simulink model "autoland_control"  (Simulink 8.4)
settings: Solver=FixedStepDiscrete  StartTime=0.0  StopTime=20.0  FixedStep=SampleTime  RelTol=1e-3
undefined symbols (not defined in the file or in its folder): AC, approach_sinkrate, approach_speed, autoland_flag, autothrottle_gains, engage_flare, flare_timeconstant, landing_sinkrate, landing_speed, SampleTime, sinkrate, sinkrate_gains, theta_sat, TrimCondition
libraries: Actuator_Lib x2, simulink x2, Controller_Lib x1
settings Model: Creator=austinmurch  LastModifiedBy=PC
settings OptimizationCC: InlineParams=on  SimCompilerOptimization=On
settings HardwareCC: ProdLargestAtomicInteger=Long  ProdLargestAtomicFloat=Double  ProdIntDivRoundTo=Zero  ProdEndianess=BigEndian  ProdHWDeviceType=Freescale->32-bit PowerPC
settings RTWCC: GenCodeOnly=on  GenerateMakefile=off  CustomSourceCode="#include \"../../../Software/FlightCode/control/rtw_grt_control.c\""

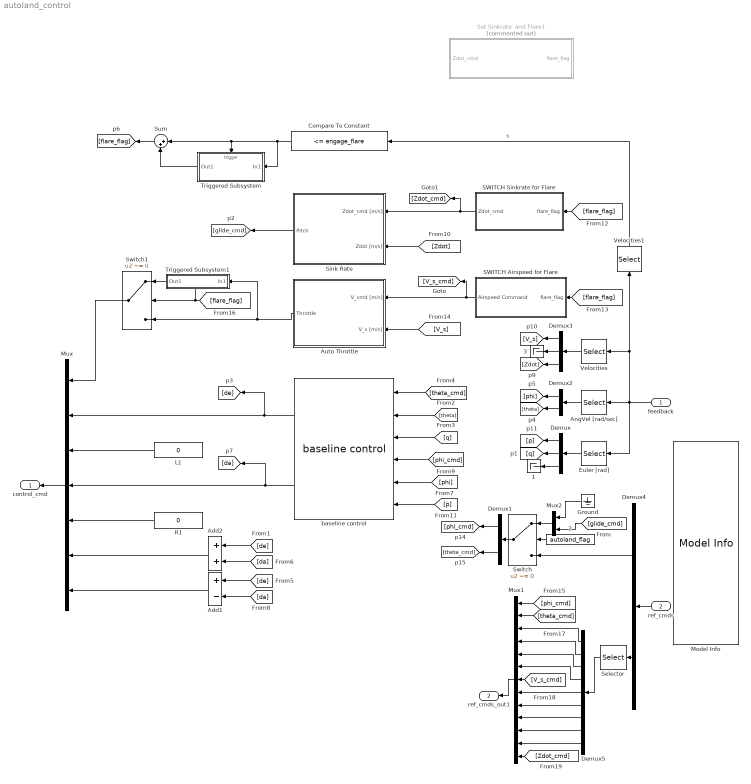
== system autoland_control ==
  feedback : Inport
  ref_cmds : Inport  Port=2
  " 2" : Constant  Value=autoland_flag
  " 1" : Terminator
  " 3" : Terminator
  Add1 : Sum  Inputs=+-
  Add2 : Sum
  AngVel [rad/sec] : Selector  InputPortWidth=19  Indices=[1:2]
  Auto Throttle : Subsystem
  Compare To Constant : simulink/Logic and Bit Operations/Compare To Constant  relop=<=  const=engage_flare  OutDataTypeStr=boolean
  Demux : Demux  Outputs=3
  Demux1 : Demux  Outputs=2
  Demux2 : Demux  Outputs=2
  Demux3 : Demux  Outputs=3
  Demux4 : Demux  Outputs=[2 10]
  Demux5 : Demux  Outputs=9
  Euler [rad] : Selector  InputPortWidth=19  Indices=[4:6]
  Ground : Ground
  L1 : Constant  Value=0
  Model Info : simulink/Model-Wide Utilities/Model Info  Frame=on  DisplayStringWithTags=|  HorizontalTextAlignment=Center  LeftAlignmentValue=0.5  SourceBlockDiagram=autoland_control  TagMaxNumber=20
      | Ref Cmd Port Info
      | 
      | 1. phi_cmd
      | 2. theta_cmd
      | 3. psi_cmd
      | 4. p_cmd
      | 5. q_cmd
      | 6. r_cmd
      | 7. V_s_cmd
      | 8. h_cmd
      | 9. gndtrk_cmd
      | 10. aoa_cmd
      | 11. aos_cmd
      | 12. gamma_cmd
      | 13. Zdot_cmd
      | 14. signal_1
      | 15. signal_2
      | 16. signal_3
      | 17. signal_4
      | 18. signal_5
      | 19. signal_6
      | 20. signal_7
      | 21. signal_8
      | 22. signal_9
  Mux : Mux  Inputs=7
  Mux1 : Mux  Inputs=13
  Mux2 : Mux  Inputs=2
  R1 : Constant  Value=0
  SWITCH Airspeed for Flare : Subsystem
  SWITCH Sinkrate for Flare : Subsystem
  Selector : Selector  InputPortWidth=10  Indices=[1:4 6:10]
  Set Sinkrate  and Flare1 : Subsystem  Commented=on
  Sink Rate : Subsystem
  Sum : Sum  Inputs=|++
  Switch : Switch  Criteria=u2 ~= 0
  Switch1 : Switch  Criteria=u2 ~= 0
  Triggered Subsystem : Subsystem  TreatAsAtomicUnit=on
  Triggered Subsystem1 : Subsystem  TreatAsAtomicUnit=on
  Velocities : Selector  InputPortWidth=19  Indices=[11,17,19]
  Velocities1 : Selector  InputPortWidth=19  Indices=[10]
  baseline control : Controller_Lib/baseline control  pitch=pitch_gains  roll=roll_gains
  control_cmd : Outport
  ref_cmds_out1 : Outport  Port=2
  wires:
  Demux/1 -> [p]
  Demux/2 -> [q]
  Demux/3 -> " 1"/1
  feedback/1 -> Velocities1/1, Velocities/1, AngVel [rad/sec]/1, Euler [rad]/1
  Demux2/2 -> [theta]
  Demux2/1 -> [phi]
  Mux/1 -> control_cmd/1
  Euler [rad]/1 -> Demux/1
  AngVel [rad/sec]/1 -> Demux2/1
  [q] -> baseline control/3
  [theta] -> baseline control/2
  [theta_cmd] -> baseline control/1
  [p] -> baseline control/6
  baseline control/1 -> [de], Mux/2
  L1/1 -> Mux/3
  [phi_cmd] -> baseline control/4
  [phi] -> baseline control/5
  R1/1 -> Mux/5
  Add2/1 -> Mux/6
  Add1/1 -> Mux/7
  [de] -> Add2/1
  [de] -> Add1/1
  [da] -> Add2/2
  [da] -> Add1/2
  baseline control/2 -> [da], Mux/4
  [V_s] -> Auto Throttle/2(V_s [m/s])
  [Zdot] -> Sink Rate/2(Zdot [m/s])
  SWITCH Airspeed for Flare/1(Airspeed Command) -> Auto Throttle/1(V_cmd [m/s]), [V_s_cmd]
  Sink Rate/1(Pitch) -> [glide_cmd]
  Auto Throttle/1(Throttle) -> Triggered Subsystem1/1(In1), Switch1/3
  Velocities/1 -> Demux3/1
  Demux3/1 -> [V_s]
  Demux3/3 -> [Zdot]
  Demux3/2 -> " 3"/1
  Mux1/1 -> ref_cmds_out1/1
  [phi_cmd] -> Mux1/1
  Demux4/2 -> Selector/1
  [theta_cmd] -> Mux1/2
  Demux4/1 -> Switch/3
  Switch/1 -> Demux1/1
  " 2"/1 -> Switch/2
  [glide_cmd] -> Mux2/2
  ref_cmds/1 -> Demux4/1
  SWITCH Sinkrate for Flare/1(Zdot_cmd) -> [Zdot_cmd], Sink Rate/1(Zdot_cmd [m/s])
  Compare To Constant/1 -> Triggered Subsystem/Trigger, Sum/1, Triggered Subsystem/1(In1)
  Triggered Subsystem/1(Out1) -> Sum/2
  Sum/1 -> [flare_flag]
  Velocities1/1 -> Compare To Constant/1  "h"
  [flare_flag] -> SWITCH Sinkrate for Flare/1(flare_flag)
  Triggered Subsystem1/1(Out1) -> Switch1/1
  [flare_flag] -> Triggered Subsystem1/Trigger, Switch1/2
  Switch1/1 -> Mux/1
  Demux1/1 -> [phi_cmd]
  Demux1/2 -> [theta_cmd]
  Mux2/1 -> Switch/1
  Ground/1 -> Mux2/1
  [flare_flag] -> SWITCH Airspeed for Flare/1(flare_flag)
  Selector/1 -> Demux5/1
  Demux5/1 -> Mux1/3
  Demux5/2 -> Mux1/4
  Demux5/3 -> Mux1/5
  Demux5/4 -> Mux1/6
  Demux5/5 -> Mux1/8
  Demux5/6 -> Mux1/9
  Demux5/7 -> Mux1/10
  Demux5/8 -> Mux1/11
  Demux5/9 -> Mux1/12
  [V_s_cmd] -> Mux1/7
  [Zdot_cmd] -> Mux1/13

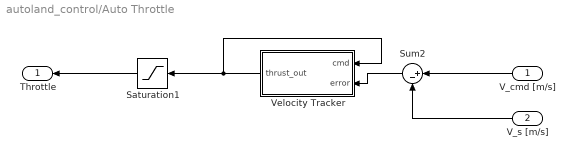
== system autoland_control/Auto Throttle ==
  V_cmd [m/s] : Inport
  V_s [m/s] : Inport  Port=2
  Saturation1 : Saturate  UpperLimit=AC.Actuator.throttle.PosLim-TrimCondition.Inputs.Throttle  LowerLimit=AC.Actuator.throttle.NegLim-TrimCondition.Inputs.Throttle  SampleTime=SampleTime
  Sum2 : Sum  Inputs=|+-  SampleTime=SampleTime
  Velocity Tracker : Subsystem
  Throttle : Outport
  wires:
  Velocity Tracker/1(thrust_out) -> Velocity Tracker/1(cmd), Saturation1/1
  V_cmd [m/s]/1 -> Sum2/1
  V_s [m/s]/1 -> Sum2/2
  Saturation1/1 -> Throttle/1
  Sum2/1 -> Velocity Tracker/2(error)

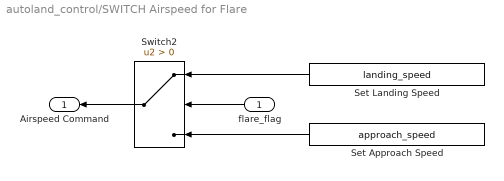
== system autoland_control/SWITCH Airspeed for Flare ==
  flare_flag : Inport
  Set Approach Speed : Constant  Value=approach_speed
  Set Landing Speed : Constant  Value=landing_speed
  Switch2 : Switch  Criteria=u2 > Threshold
  Airspeed Command : Outport
  wires:
  Set Approach Speed/1 -> Switch2/3
  flare_flag/1 -> Switch2/2
  Switch2/1 -> Airspeed Command/1
  Set Landing Speed/1 -> Switch2/1

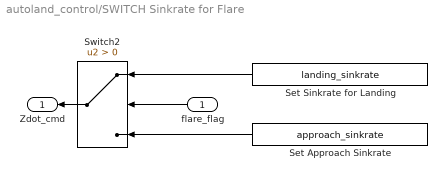
== system autoland_control/SWITCH Sinkrate for Flare ==
  flare_flag : Inport
  Set Approach Sinkrate : Constant  Value=approach_sinkrate
  Set Sinkrate for Landing : Constant  Value=landing_sinkrate
  Switch2 : Switch  Criteria=u2 > Threshold
  Zdot_cmd : Outport
  wires:
  Set Sinkrate for Landing/1 -> Switch2/1
  Switch2/1 -> Zdot_cmd/1
  flare_flag/1 -> Switch2/2
  Set Approach Sinkrate/1 -> Switch2/3

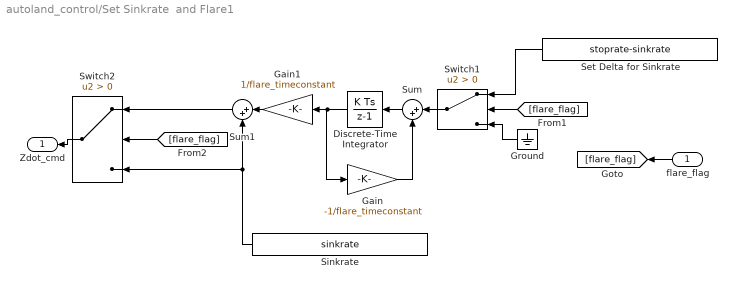
== system autoland_control/Set Sinkrate  and Flare1 ==
  flare_flag : Inport
  Discrete-Time Integrator : DiscreteIntegrator  InitialConditionSetting=State (most efficient)  SampleTime=SampleTime
  Gain : Gain  Gain=-1/flare_timeconstant
  Gain1 : Gain  Gain=1/flare_timeconstant
  Ground : Ground
  Set Delta for Sinkrate : Constant  Value=stoprate-sinkrate
  Sinkrate : Constant  Value=sinkrate
  Sum : Sum  Inputs=|++
  Sum1 : Sum  Inputs=|++
  Switch1 : Switch  Criteria=u2 > Threshold
  Switch2 : Switch  Criteria=u2 > Threshold
  Zdot_cmd : Outport
  wires:
  Sinkrate/1 -> Switch2/3, Sum1/2
  [flare_flag] -> Switch2/2
  [flare_flag] -> Switch1/2
  flare_flag/1 -> [flare_flag]
  Switch2/1 -> Zdot_cmd/1
  Sum1/1 -> Switch2/1
  Discrete-Time Integrator/1 -> Gain1/1, Gain/1
  Sum/1 -> Discrete-Time Integrator/1
  Gain1/1 -> Sum1/1
  Switch1/1 -> Sum/1
  Set Delta for Sinkrate/1 -> Switch1/1
  Ground/1 -> Switch1/3
  Gain/1 -> Sum/2

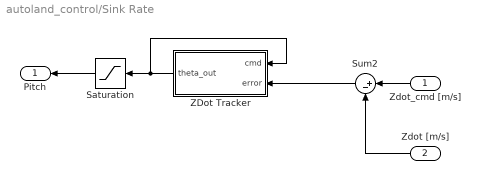
== system autoland_control/Sink Rate ==
  Zdot_cmd [m/s] : Inport
  Zdot [m/s] : Inport  Port=2
  Saturation : Saturate  UpperLimit=theta_sat/180*pi  LowerLimit=-theta_sat/180*pi
  Sum2 : Sum  Inputs=|+-  SampleTime=SampleTime
  ZDot Tracker : Subsystem
  Pitch : Outport
  wires:
  Zdot [m/s]/1 -> Sum2/2
  Sum2/1 -> ZDot Tracker/2(error)
  Zdot_cmd [m/s]/1 -> Sum2/1
  ZDot Tracker/1(theta_out) -> ZDot Tracker/1(cmd), Saturation/1
  Saturation/1 -> Pitch/1

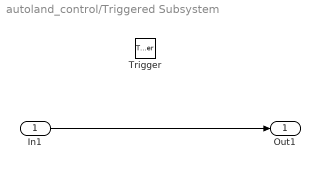
== system autoland_control/Triggered Subsystem ==
  In1 : Inport
  Trigger : TriggerPort
  Out1 : Outport
  wires:
  In1/1 -> Out1/1

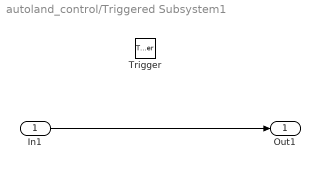
== system autoland_control/Triggered Subsystem1 ==
  In1 : Inport
  Trigger : TriggerPort
  Out1 : Outport
  wires:
  In1/1 -> Out1/1

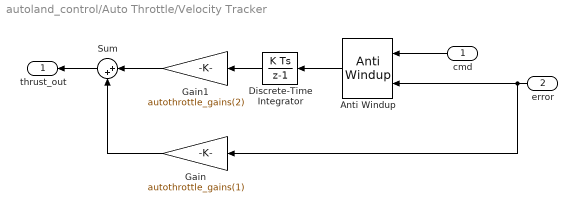
== system autoland_control/Auto Throttle/Velocity Tracker ==
  cmd : Inport
  error : Inport  Port=2
  Anti Windup : Actuator_Lib/Anti Windup  MAX_DEF=AC.Actuator.throttle.PosLim-TrimCondition.Inputs.Throttle  MIN_DEF=AC.Actuator.throttle.NegLim-TrimCondition.Inputs.Throttle  gain_sign=on
  Discrete-Time Integrator : DiscreteIntegrator  SampleTime=SampleTime
  Gain : Gain  Gain=autothrottle_gains(1)
  Gain1 : Gain  Gain=autothrottle_gains(2)
  Sum : Sum  Inputs=|++
  thrust_out : Outport
  wires:
  Discrete-Time Integrator/1 -> Gain1/1
  Gain1/1 -> Sum/1
  Sum/1 -> thrust_out/1
  Gain/1 -> Sum/2
  error/1 -> Anti Windup/2, Gain/1
  cmd/1 -> Anti Windup/1
  Anti Windup/1 -> Discrete-Time Integrator/1

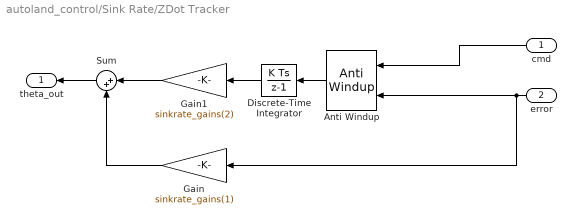
== system autoland_control/Sink Rate/ZDot Tracker ==
  cmd : Inport
  error : Inport  Port=2
  Anti Windup : Actuator_Lib/Anti Windup  MAX_DEF=theta_sat/180*pi  MIN_DEF=-theta_sat/180*pi  gain_sign=off
  Discrete-Time Integrator : DiscreteIntegrator  SampleTime=SampleTime
  Gain : Gain  Gain=sinkrate_gains(1)
  Gain1 : Gain  Gain=sinkrate_gains(2)
  Sum : Sum  Inputs=|++
  theta_out : Outport
  wires:
  Discrete-Time Integrator/1 -> Gain1/1
  Gain1/1 -> Sum/1
  Sum/1 -> theta_out/1
  Gain/1 -> Sum/2
  error/1 -> Anti Windup/2, Gain/1
  cmd/1 -> Anti Windup/1
  Anti Windup/1 -> Discrete-Time Integrator/1
